simulink model "HarmOscillatorModel"  (R2023b)
settings: Solver=ode4  StartTime=0.0  StopTime=tf  FixedStep=ts  RelTol=1e-3
values from neighbouring files (symbols this model uses):
  b = 1.5    [HarmonicOscillator.m]
  F = 300    [HarmonicOscillator.m]
  Fstep = 0.5    [HarmonicOscillator.m]
  k = 15.0    (= 15)    [HarmonicOscillator.m]
  Kd = 0    [HarmonicOscillator.m]
  Ki = 0    [HarmonicOscillator.m]
  Kp = 0    [HarmonicOscillator.m]
  m = 10.0    (= 10)    [HarmonicOscillator.m]
  V0 = 0    [HarmonicOscillator.m]
  X0 = 0    [HarmonicOscillator.m]
  xgoal = 3    [HarmonicOscillator.m]
settings Model: Creator=Owner  LastModifiedBy=billy
settings DataIOCC: ReturnWorkspaceOutputs=off

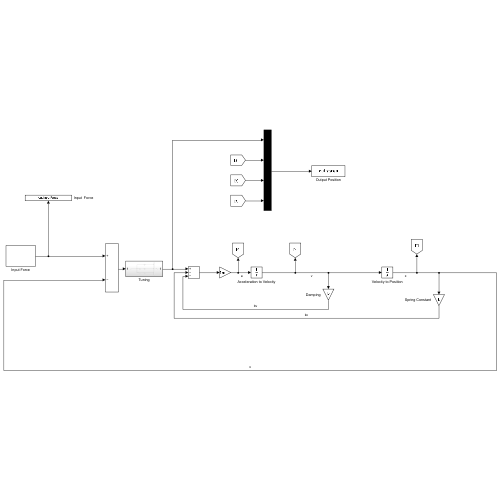
[thumbnail: Simulink's stored preview of the top-level diagram]
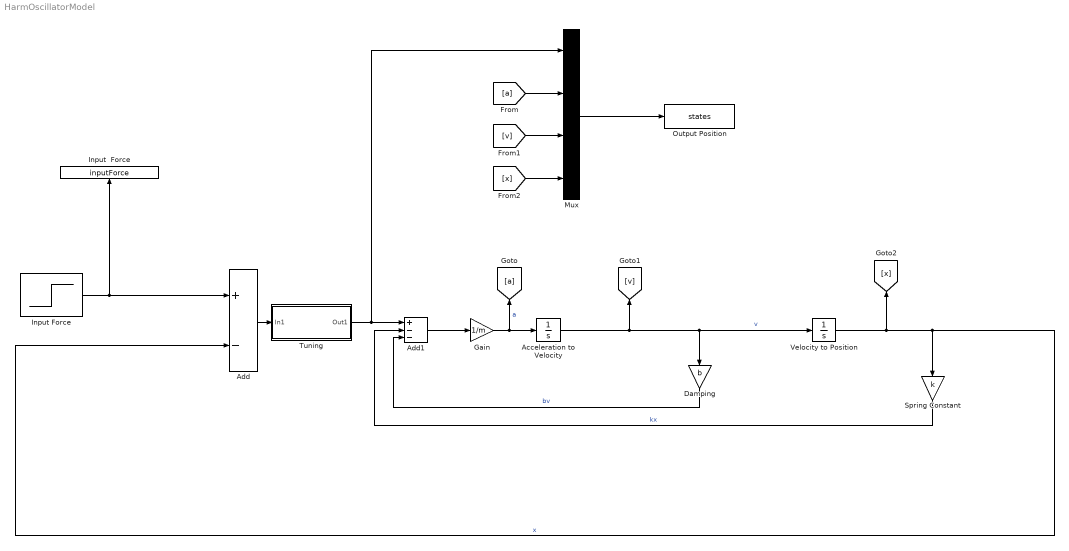
== system HarmOscillatorModel ==
  Acceleration to Velocity : Integrator  InitialCondition=V0
  Add : Sum  Inputs=+-
  Add1 : Sum  Inputs=+--
  Damping : Gain  Gain=b
  Gain : Gain  Gain=1/m
  Input  Force : ToWorkspace  VariableName=inputForce  SaveFormat=Timeseries  SampleTime=-1
  Input Force : Step  Time=Fstep  Before=F  After=xgoal  SampleTime=0
  Mux : Mux
  Output Position : ToWorkspace  VariableName=states  SampleTime=-1
  Spring Constant : Gain  Gain=k
  Tuning : Subsystem
  Velocity to Position : Integrator  InitialCondition=X0
  wires:
  Input Force/1 -> Add/1, Input  Force/1
  Velocity to Position/1 -> Add/2, Spring Constant/1, [x]  "x"
  Add/1 -> Tuning/1(In1)
  Tuning/1(Out1) -> Mux/1, Add1/1
  Gain/1 -> Acceleration to Velocity/1, [a]  "a"
  Acceleration to Velocity/1 -> Velocity to Position/1, Damping/1, [v]  "v"
  Damping/1 -> Add1/3  "bv"
  Add1/1 -> Gain/1
  Spring Constant/1 -> Add1/2  "kx"
  [a] -> Mux/2
  [v] -> Mux/3
  [x] -> Mux/4
  Mux/1 -> Output Position/1

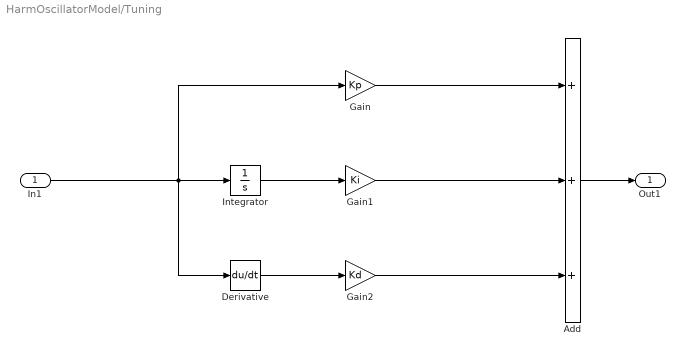
== system HarmOscillatorModel/Tuning ==
  In1 : Inport
  Add : Sum  Inputs=+++
  Derivative : Derivative
  Gain : Gain  Gain=Kp
  Gain1 : Gain  Gain=Ki
  Gain2 : Gain  Gain=Kd
  Integrator : Integrator
  Out1 : Outport
  wires:
  In1/1 -> Derivative/1, Integrator/1, Gain/1
  Integrator/1 -> Gain1/1
  Derivative/1 -> Gain2/1
  Gain2/1 -> Add/3
  Gain1/1 -> Add/2
  Gain/1 -> Add/1
  Add/1 -> Out1/1
